simulink model "Position_Control"  (R2016a)
settings: Solver=VariableStepAuto  StartTime=0.0  StopTime=10.0  RelTol=1e-3
settings Model: Creator=dell  LastModifiedBy=dell

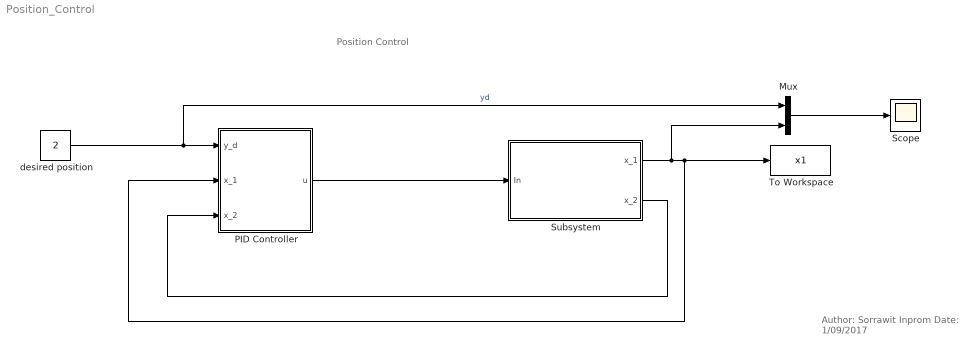
== system Position_Control ==
  note: Author: Sorrawit Inprom
      | Date: 1/09/2017
  note: Position Control
  Mux : Mux  Inputs=2
  PID Controller : Subsystem
  Scope : Scope
  Subsystem : Subsystem
  To Workspace : ToWorkspace  VariableName=x1  SaveFormat=Timeseries  SampleTime=-1
  desired position : Constant  Value=2
  wires:
  desired position/1 -> Mux/1, PID Controller/1(y_d)  "yd"
  Subsystem/2(x_2) -> PID Controller/3(x_2)
  PID Controller/1(u) -> Subsystem/1(In)
  Mux/1 -> Scope/1
  Subsystem/1(x_1) -> To Workspace/1, PID Controller/2(x_1), Mux/2

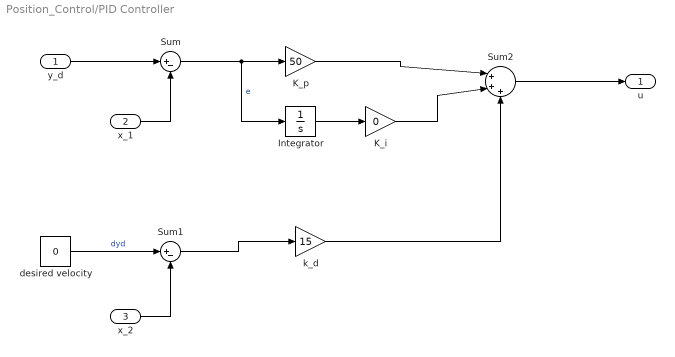
== system Position_Control/PID Controller ==
  y_d : Inport
  x_1 : Inport  Port=2
  x_2 : Inport  Port=3
  Integrator : Integrator
  K_i : Gain  Gain=0
  K_p : Gain  Gain=50
  Sum : Sum  Inputs=|+-
  Sum1 : Sum  Inputs=|+-
  Sum2 : Sum  Inputs=|+++
  desired velocity : Constant  Value=0
  k_d : Gain  Gain=15
  u : Outport
  wires:
  x_1/1 -> Sum/2
  Integrator/1 -> K_i/1
  desired velocity/1 -> Sum1/1  "dyd"
  x_2/1 -> Sum1/2
  y_d/1 -> Sum/1
  Sum/1 -> Integrator/1, K_p/1  "e"
  Sum1/1 -> k_d/1
  K_i/1 -> Sum2/2
  Sum2/1 -> u/1
  k_d/1 -> Sum2/3
  K_p/1 -> Sum2/1

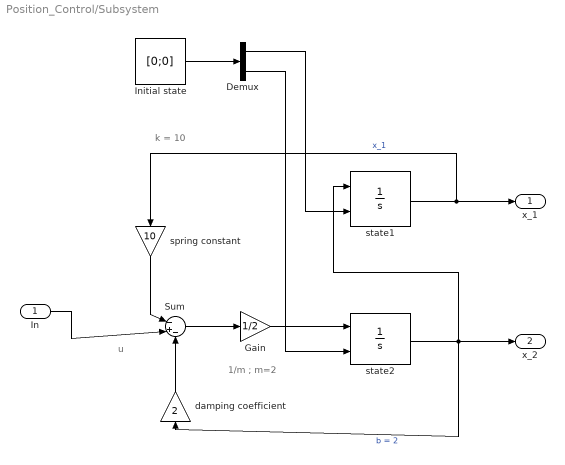
== system Position_Control/Subsystem ==
  note: k = 10
  note: u
  note: 1/m ; m=2
  In : Inport
  Demux : Demux  Outputs=2
  Gain : Gain  Gain=1/2
  Initial state : Constant  Value=[0;0]
  Sum : Sum  Inputs=|-+-
  damping coefficient : Gain  Gain=2
  spring constant : Gain  Gain=10
  state1 : Integrator  InitialConditionSource=external  ContinuousStateAttributes='position'
  state2 : Integrator  InitialConditionSource=external  ContinuousStateAttributes='velocity'
  x_1 : Outport
  x_2 : Outport  Port=2
  wires:
  Gain/1 -> state2/1
  state2/1 -> damping coefficient/1, x_2/1, state1/1  "b = 2"
  damping coefficient/1 -> Sum/3
  Sum/1 -> Gain/1
  spring constant/1 -> Sum/1
  In/1 -> Sum/2
  state1/1 -> x_1/1, spring constant/1  "x_1"
  Initial state/1 -> Demux/1
  Demux/1 -> state1/2
  Demux/2 -> state2/2
